simulink model "InductionCookerStateFlow_HarnessButtonS2"  (R2023a)
settings: Solver=FixedStepDiscrete  StartTime=0.0  StopTime=200  FixedStep=0.1  RelTol=1e-3  EnableMultiTasking=on
settings Model: Creator=anton  LastModifiedBy=anton
settings SolverCC: AlgebraicLoopSolver=TrustRegion  AutoInsertRateTranBlk=on
settings DataIOCC: LimitDataPoints=on
settings OptimizationCC: LifeSpan=inf
settings DebuggingCC: UnconnectedInputMsg=warning  UnconnectedOutputMsg=warning  UnconnectedLineMsg=warning  AllowSymbolicDim=off  SFUnexpectedBacktrackingDiag=warning  SFNoUnconditionalDefaultTransitionDiag=warning  SFExecutionAtInitializationDiag=none  ArithmeticOperatorsInVariantConditions=warning
settings ModelReferenceCC: EnableRefExpFcnMdlSchedulingChecks=on
settings SFSimCC: SimUseLocalCustomCode=off  CustomCodeUndefinedFunction=UseInterfaceOnly
settings RTWCC: RTWUseLocalCustomCode=off  DLArmComputeVersion=19.05
settings CodeAppCC: StateflowObjectComments=on
settings GRTTargetCC: TargetLangStandard=C89/C90 (ANSI)
settings ConfigComp: CovEnable=on  RecordCoverage=on  CovMetricSettings=dw  CovSaveCumulativeToWorkspaceVar=on  CovSaveSingleToWorkspaceVar=on  CovModelRefEnable=on

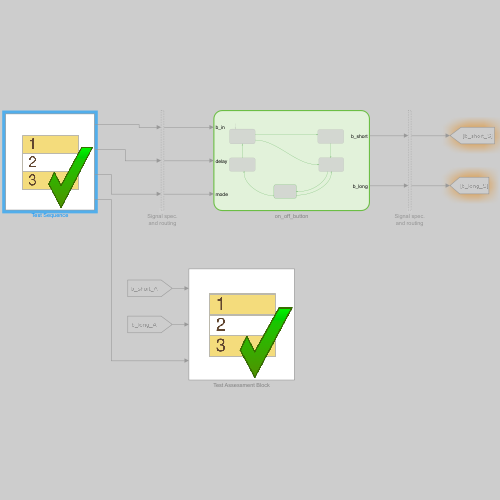
[thumbnail: Simulink's stored preview of the top-level diagram]
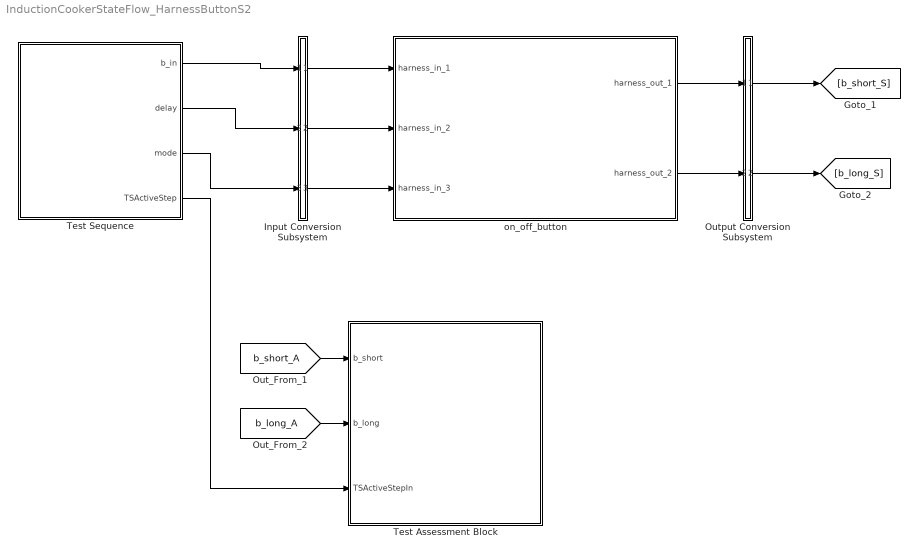
== system InductionCookerStateFlow_HarnessButtonS2 ==
  Input Conversion Subsystem : Subsystem  Tag=__SLT_ICS__  Description=|
      | Signal spec.
      | and routing
      settings: AttributesFormatString=%<Description>
  Output Conversion Subsystem : Subsystem  Tag=__SLT_OCS__  Description=|
      | Signal spec.
      | and routing
      settings: AttributesFormatString=%<Description>
  Test Assessment Block : Test Sequence  Tag=__SLT_ASMT__  TreatAsAtomicUnit=on
  Test Sequence : Test Sequence  TreatAsAtomicUnit=on
  on_off_button : Subsystem  Tag=__SL_testing_harness_stub_
  wires:
  [b_short_A] -> Test Assessment Block/1(b_short)
  [b_long_A] -> Test Assessment Block/2(b_long)
  Test Sequence/1(b_in) -> Input Conversion Subsystem/1(Inport_1)
  Test Sequence/2(delay) -> Input Conversion Subsystem/2(Inport_2)
  Test Sequence/3(mode) -> Input Conversion Subsystem/3(Inport_3)
  Output Conversion Subsystem/1(Outport_1) -> [b_short_S]
  Output Conversion Subsystem/2(Outport_2) -> [b_long_S]
  Test Sequence/4(TSActiveStep) -> Test Assessment Block/3(TSActiveStepIn)
  on_off_button/1(harness_out_1) -> Output Conversion Subsystem/1(Inport_1)
  on_off_button/2(harness_out_2) -> Output Conversion Subsystem/2(Inport_2)
  Input Conversion Subsystem/1(Outport_1) -> on_off_button/1(harness_in_1)
  Input Conversion Subsystem/2(Outport_2) -> on_off_button/2(harness_in_2)
  Input Conversion Subsystem/3(Outport_3) -> on_off_button/3(harness_in_3)

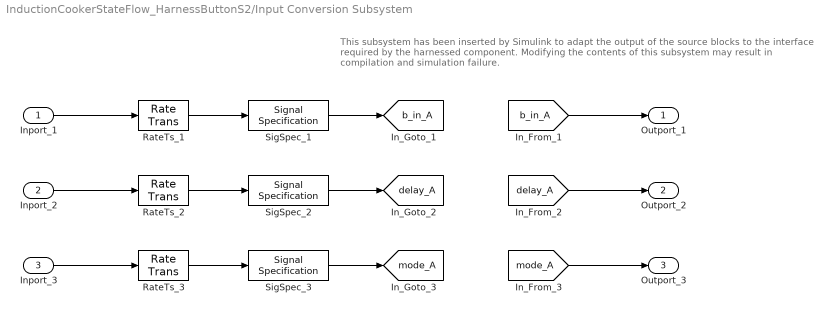
== system InductionCookerStateFlow_HarnessButtonS2/Input Conversion Subsystem ==
  note: This subsystem has been inserted by Simulink to adapt the output of the source blocks to the interface required by the harnessed component.
      |  Modifying the contents of this subsystem may result in compilation and simulation failure.
  Inport_1 : Inport
  Inport_2 : Inport  Port=2
  Inport_3 : Inport  Port=3
  RateTs_1 : RateTransition  OutPortSampleTime=0.1
  RateTs_2 : RateTransition  OutPortSampleTime=[-1, 0]
  RateTs_3 : RateTransition  OutPortSampleTime=[-1, 0]
  SigSpec_1 : SignalSpecification  OutDataTypeStr=boolean  Dimensions=[1]  SampleTime=0.1
  SigSpec_2 : SignalSpecification  OutDataTypeStr=double  Dimensions=[1]  SampleTime=[-1, 0]
  SigSpec_3 : SignalSpecification  OutDataTypeStr=uint8  Dimensions=[1]  SampleTime=[-1, 0]
  Outport_1 : Outport
  Outport_2 : Outport  Port=2
  Outport_3 : Outport  Port=3
  tag scope: b_in_A=global, delay_A=global, mode_A=global
  wires:
  [b_in_A] -> Outport_1/1
  SigSpec_1/1 -> [b_in_A]
  RateTs_1/1 -> SigSpec_1/1
  Inport_1/1 -> RateTs_1/1
  [delay_A] -> Outport_2/1
  SigSpec_2/1 -> [delay_A]
  RateTs_2/1 -> SigSpec_2/1
  Inport_2/1 -> RateTs_2/1
  [mode_A] -> Outport_3/1
  SigSpec_3/1 -> [mode_A]
  RateTs_3/1 -> SigSpec_3/1
  Inport_3/1 -> RateTs_3/1

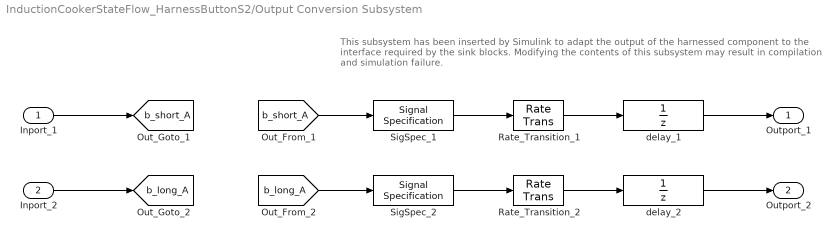
== system InductionCookerStateFlow_HarnessButtonS2/Output Conversion Subsystem ==
  note: This subsystem has been inserted by Simulink to adapt the output of the harnessed component to the interface required by the sink blocks.
      |  Modifying the contents of this subsystem may result in compilation and simulation failure.
  Inport_1 : Inport
  Inport_2 : Inport  Port=2
  Rate_Transition_1 : RateTransition  OutPortSampleTimeOpt=Inherit
  Rate_Transition_2 : RateTransition  OutPortSampleTimeOpt=Inherit
  SigSpec_1 : SignalSpecification  OutDataTypeStr=boolean  Dimensions=[1]  SampleTime=0.1
  SigSpec_2 : SignalSpecification  OutDataTypeStr=boolean  Dimensions=[1]  SampleTime=0.1
  delay_1 : UnitDelay  SampleTime=-1
  delay_2 : UnitDelay  SampleTime=-1
  Outport_1 : Outport
  Outport_2 : Outport  Port=2
  tag scope: b_long_A=global, b_short_A=global
  wires:
  Inport_1/1 -> [b_short_A]
  [b_short_A] -> SigSpec_1/1
  SigSpec_1/1 -> Rate_Transition_1/1
  Rate_Transition_1/1 -> delay_1/1
  delay_1/1 -> Outport_1/1
  Inport_2/1 -> [b_long_A]
  [b_long_A] -> SigSpec_2/1
  SigSpec_2/1 -> Rate_Transition_2/1
  Rate_Transition_2/1 -> delay_2/1
  delay_2/1 -> Outport_2/1

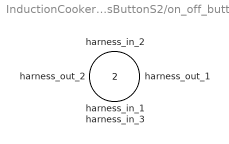
== system InductionCookerStateFlow_HarnessButtonS2/on_off_button ==
  harness_in_1 : Inport
  harness_in_2 : Inport  Port=2
  harness_in_3 : Inport  Port=3
  harness_out_1 : Outport
  harness_out_2 : Outport  Port=2

== stateflow chart InductionCookerStateFlow_HarnessButtonS2/Test Assessment Block ==
  state Scenario_1
    state Run
      state VerifyInitWait_S2
        verify(b_long & b_short);
      state VerifyInit_S2
        verify(b_long & b_short);
      state VerifyButtonShortPressed_S2
        verify(b_short & b_long);
      state VerifyButtonShortPressedWait_S2
        verify(b_short & b_long);
      state VerifyButtonFirstReleased_S2
        verify(b_short & b_long);
      state VerifyButtonFirstLongPressed_S2
        state VerifyButtonFirstLongPressed_1_S2
          verify(b_short & b_long)
        state VerifyButtonFirstLongPressed_2_S2
          verify(b_short & ~b_long)
        (default) -> VerifyButtonFirstLongPressed_1_S2
        VerifyButtonFirstLongPressed_1_S2 -> VerifyButtonFirstLongPressed_2_S2 : [
            | after(1,sec)
            | ]
      state VerifyButtonSecondLongPressed_S2
        verify(b_long & b_short);
      state VerifyButtonSecondLongPressedWait_S2
        verify(b_long & b_short);
      state VerifyButtonSecondReleased_S2
        verify(b_long & b_short);
      state step_1_2
      (default) -> (junction 245)
      Run -> (junction 245)
      (junction 245) -> (junction 246) [order 1] : [TSActiveStepIn == TSActiveStepEnumButton.InitWait_S2
          | ]
      (junction 246) -> VerifyInitWait_S2 [order 1] : [~in(Scenario_1.Run.VerifyInitWait_S2)]
      (junction 245) -> (junction 382) [order 2]
      (junction 246) -> (junction 249) [order 2]
      (junction 382) -> (junction 383) [order 1] : [TSActiveStepIn == TSActiveStepEnumButton.Init_S2
          | ]
      (junction 383) -> VerifyInit_S2 [order 1] : [~in(Scenario_1.Run.VerifyInit_S2)]
      (junction 382) -> (junction 270) [order 2]
      (junction 383) -> (junction 386) [order 2]
      (junction 270) -> (junction 271) [order 1] : [TSActiveStepIn == TSActiveStepEnumButton.ButtonShortPressed_S2
          | ]
      (junction 271) -> VerifyButtonShortPressed_S2 [order 1] : [~in(Scenario_1.Run.VerifyButtonShortPressed_S2)]
      (junction 270) -> (junction 373) [order 2]
      (junction 271) -> (junction 274) [order 2]
      (junction 373) -> (junction 374) [order 1] : [TSActiveStepIn == TSActiveStepEnumButton.ButtonShortPressedWait_S2
          | ]
      (junction 374) -> VerifyButtonShortPressedWait_S2 [order 1] : [~in(Scenario_1.Run.VerifyButtonShortPressedWait_S2)]
      (junction 373) -> (junction 278) [order 2]
      (junction 374) -> (junction 377) [order 2]
      (junction 278) -> (junction 279) [order 1] : [TSActiveStepIn == TSActiveStepEnumButton.ButtonFirstReleased_S2
          | ]
      (junction 279) -> VerifyButtonFirstReleased_S2 [order 1] : [~in(Scenario_1.Run.VerifyButtonFirstReleased_S2)]
      (junction 278) -> (junction 286) [order 2]
      (junction 279) -> (junction 282) [order 2]
      (junction 286) -> (junction 287) [order 1] : [TSActiveStepIn == TSActiveStepEnumButton.ButtonFirstLongPressed_S2
          | ]
      (junction 287) -> VerifyButtonFirstLongPressed_S2 [order 1] : [~in(Scenario_1.Run.VerifyButtonFirstLongPressed_S2)]
      (junction 286) -> (junction 309) [order 2]
      (junction 287) -> (junction 290) [order 2]
      (junction 309) -> (junction 310) [order 1] : [TSActiveStepIn == TSActiveStepEnumButton.ButtonSecondLongPressed_S2
          | ]
      (junction 310) -> VerifyButtonSecondLongPressed_S2 [order 1] : [~in(Scenario_1.Run.VerifyButtonSecondLongPressed_S2)]
      (junction 309) -> (junction 391) [order 2]
      (junction 310) -> (junction 313) [order 2]
      (junction 391) -> (junction 392) [order 1] : [TSActiveStepIn == TSActiveStepEnumButton.ButtonSecondLongPressedWait_S2
          | ]
      (junction 392) -> VerifyButtonSecondLongPressedWait_S2 [order 1] : [~in(Scenario_1.Run.VerifyButtonSecondLongPressedWait_S2)]
      (junction 391) -> (junction 318) [order 2]
      (junction 392) -> (junction 395) [order 2]
      (junction 318) -> (junction 319) [order 1] : [TSActiveStepIn == TSActiveStepEnumButton.ButtonSecondReleased_S2
          | ]
      (junction 319) -> VerifyButtonSecondReleased_S2 [order 1] : [~in(Scenario_1.Run.VerifyButtonSecondReleased_S2)]
      (junction 318) -> (junction 334) [order 2]
      (junction 319) -> (junction 322) [order 2]
      (junction 334) -> (junction 335)
      (junction 335) -> step_1_2 [order 1] : [~in(Scenario_1.Run.step_1_2)]
      (junction 335) -> (junction 338) [order 2]
    (default) -> Run
  (default) -> Scenario_1 : {assert(Active_Scenario_Index == 1,'The value of Scenario Parameter ''Active_Scenario_Index'' is not valid. Use the index of the scenario to specify it.')}
  data: b_short input boolean size=[1]; b_long input boolean size=[1]; TSActiveStepIn input; Active_Scenario_Index parameter =1

== stateflow chart InductionCookerStateFlow_HarnessButtonS2/Test Sequence ==
  settings: updateMethod=DISCRETE  sampleTime=0.1
  state Scenario_1
    state InitWait_S2
      b_in = true;
      delay = 1;
      mode = uint8(0);
      settings: description=|
          | Situazione iniziale in cui la modalità operativa
          | è (0) per coprire il caso in cui la
          | transizione sia falsa.
    state Init_S2
      b_in = true;
      delay = 1;
      mode = uint8(1);
      settings: description=|
          | Rappresenta la situazione in cui il
          | pulsante non è ancora premuto e la
          | modalità operativa selezionata (1)
          | è quella di aumento/diminuzione della
          | potenza.
    state ButtonShortPressed_S2
      b_in = false;
      delay = 1;
      mode = uint8(1);
      settings: description=|
          | Pressione del pulsante, considerando questo
          | step attivo per 0,5 secondi. Mi aspetto che il
          | livello alto del bottone non venga raggiunto
    state ButtonShortPressedWait_S2
      b_in = false;
      delay = 1;
      mode = uint8(1);
      settings: description=|
          | Pressione del pulsante per coprire il caso in cui la
          | transizione sia falsa.
    state ButtonFirstReleased_S2
      b_in = true;
      delay = 1;
      mode = uint8(1);
      settings: description=Rilascio del bottone.
    state ButtonFirstLongPressed_S2
      b_in = false;
      delay = 1;
      mode = uint8(1);
      settings: description=|
          | Pressione del pulsante per un secondo e mezzo.
          | Mi aspetto che il livello alto del pulsante venga raggiunto,
          | in quanto la pressione viene effettuata per almeno
          | 1 secondo.
    state ButtonSecondLongPressed_S2
      b_in = false;
      delay = 1;
      mode = uint8(1);
      settings: description=Catturo l'uscita b_long = PRESSED.
    state ButtonSecondLongPressedWait_S2
      b_in = false;
      delay = 1;
      mode = uint8(1);
      settings: description=|
          | Pressione del pulsante per coprire il caso in cui la
          | transizione sia falsa.
    state ButtonSecondReleased_S2
      b_in = true;
      delay = 1;
      mode = uint8(1);
      settings: description=Rilascio del bottone.
    (default) -> InitWait_S2
    Init_S2 -> ButtonShortPressed_S2 : [
        | true
        | ]
    ButtonShortPressed_S2 -> ButtonShortPressedWait_S2 : [
        | after(0.5, sec)
        | ]
    ButtonShortPressedWait_S2 -> ButtonFirstReleased_S2 : [
        | true
        | ]
    ButtonFirstReleased_S2 -> ButtonFirstLongPressed_S2 : [
        | true
        | ]
    ButtonFirstLongPressed_S2 -> ButtonSecondLongPressed_S2 : [
        | after(delay+sampleTime, sec)
        | ]
    ButtonSecondLongPressed_S2 -> ButtonSecondLongPressedWait_S2 : [
        | true
        | ]
    ButtonSecondLongPressedWait_S2 -> ButtonSecondReleased_S2 : [
        | true
        | ]
    InitWait_S2 -> Init_S2 : [
        | true
        | ]
  (default) -> Scenario_1 : {assert(Active_Scenario_Index == 1,'The value of Scenario Parameter ''Active_Scenario_Index'' is not valid. Use the index of the scenario to specify it.')}
  data: b_in output boolean size=[1]; delay output double size=[1]; mode output uint8 size=[1]; TSActiveStep output Enum: TSActiveStepEnumButton; sampleTime constant double =str2num(get_param('InductionCoockerStateFlow','FixedStep')); Active_Scenario_Index parameter =1
